simulink model "bucksim"  (R2022b)
settings: Solver=FixedStepAuto  StartTime=0.0  StopTime=0.001  FixedStep=1/(1000 * fsw)  RelTol=1e-3
values from neighbouring files (symbols this model uses):
  Don = 0.42    [answers.m]
  fsw = 10^5    (= 100000)    [answers.m]
  L = 1e-4    (= 0.0001)    [answers.m]
  R = 10    [answers.m]
  Vin = 12    [answers.m]
undefined symbols (not defined in the file or in its folder): C
libraries: simulink x3
settings Model: Creator=gabriel5leonard  LastModifiedBy=gabriel5leonard

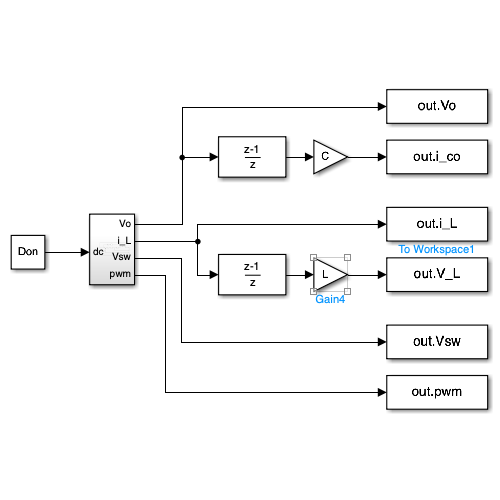
[thumbnail: Simulink's stored preview of the top-level diagram]
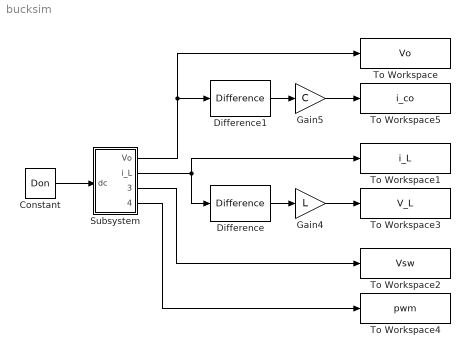
== system bucksim ==
  Constant : Constant  Value=Don
  Difference : simulink/Discrete/Difference  ICPrevInput=0.0  OutMin=[]  OutMax=[]  OutDataType=fixdt(1, 16)  OutScaling=2^-10  DoSatur=off
  Difference1 : simulink/Discrete/Difference  ICPrevInput=0.0  OutMin=[]  OutMax=[]  OutDataType=fixdt(1, 16)  OutScaling=2^-10  DoSatur=off
  Gain4 : Gain  Gain=L
  Gain5 : Gain  Gain=C
  Subsystem : Subsystem
  To Workspace : ToWorkspace  VariableName=Vo  SaveFormat=Structure With Time  SampleTime=-1
  To Workspace1 : ToWorkspace  VariableName=i_L  SaveFormat=Structure With Time  SampleTime=-1
  To Workspace2 : ToWorkspace  VariableName=Vsw  SaveFormat=Structure With Time  SampleTime=-1
  To Workspace3 : ToWorkspace  VariableName=V_L  SaveFormat=Structure With Time  SampleTime=-1
  To Workspace4 : ToWorkspace  VariableName=pwm  SaveFormat=Structure With Time  SampleTime=-1
  To Workspace5 : ToWorkspace  VariableName=i_co  SaveFormat=Structure With Time  SampleTime=-1
  wires:
  Constant/1 -> Subsystem/1(dc)
  Subsystem/3(Vsw) -> To Workspace2/1
  Subsystem/4(pwm) -> To Workspace4/1
  Subsystem/1(Vo) -> To Workspace/1, Difference1/1
  Gain5/1 -> To Workspace5/1
  Gain4/1 -> To Workspace3/1
  Subsystem/2(i_L) -> Difference/1, To Workspace1/1
  Difference1/1 -> Gain5/1
  Difference/1 -> Gain4/1

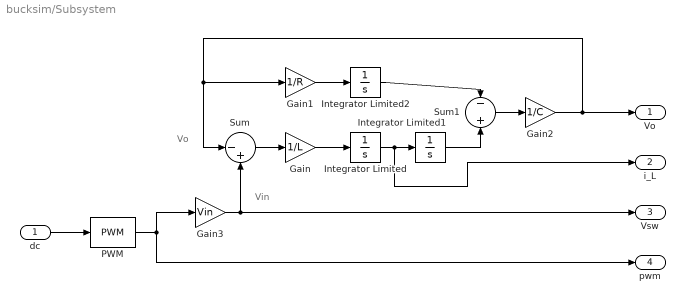
== system bucksim/Subsystem ==
  note: Vin
  note: Vo
  dc : Inport
  Gain : Gain  Gain=1/L
  Gain1 : Gain  Gain=1/R
  Gain2 : Gain  Gain=1/C
  Gain3 : Gain  Gain=Vin
  Integrator Limited : Integrator  LimitOutput=on  UpperSaturationLimit=10000  LowerSaturationLimit=0
  Integrator Limited1 : Integrator  LimitOutput=on  UpperSaturationLimit=10000  LowerSaturationLimit=0
  Integrator Limited2 : Integrator  LimitOutput=on  UpperSaturationLimit=10000  LowerSaturationLimit=0
  PWM : simulink/Discontinuities/PWM  DisableCoverage=on  Period=1/fsw  InitialDelay=0  DisallowZeroDutyCycle=off  RunAtFixedTimeIntervals=on  SampleTime=1/(1000*fsw)
  Sum : Sum  Inputs=|-+
  Sum1 : Sum  Inputs=-|+
  Vo : Outport
  i_L : Outport  Port=2
  Vsw : Outport  Port=3
  pwm : Outport  Port=4
  wires:
  dc/1 -> PWM/1
  Gain/1 -> Integrator Limited/1
  Sum/1 -> Gain/1
  Sum1/1 -> Gain2/1
  Integrator Limited/1 -> Integrator Limited1/1, i_L/1
  Integrator Limited2/1 -> Sum1/1
  Gain3/1 -> Vsw/1, Sum/2
  Integrator Limited1/1 -> Sum1/2
  PWM/1 -> Gain3/1, pwm/1
  Gain1/1 -> Integrator Limited2/1
  Gain2/1 -> Vo/1, Sum/1, Gain1/1
